simulink model "WR_UDE"  (R2020a)
settings: Solver=ode4  StartTime=0.0  StopTime=tstop  FixedStep=tstep  RelTol=1e-3
values from neighbouring files (symbols this model uses):
  eic = xic - xmic    [data.m]
  K = dlqr(F_n, G_n, Q, R)    [data.m]
  Ts = 0.01    [data.m]
  udic = (-Ts/T)*pinv(G_n)*eic    [data.m]
  xhat_ic = [pi/9; 0]    [data.m]
  xic = [pi/9; 0]    [data.m]
  xmic = [0; 0]    [data.m]
settings Model: Creator=Ram Padmanabhan  LastModifiedBy=Maithili Shetty
settings DataIOCC: SaveOutput=off  SignalLogging=off  DSMLogging=off  SaveTime=off  ReturnWorkspaceOutputs=off

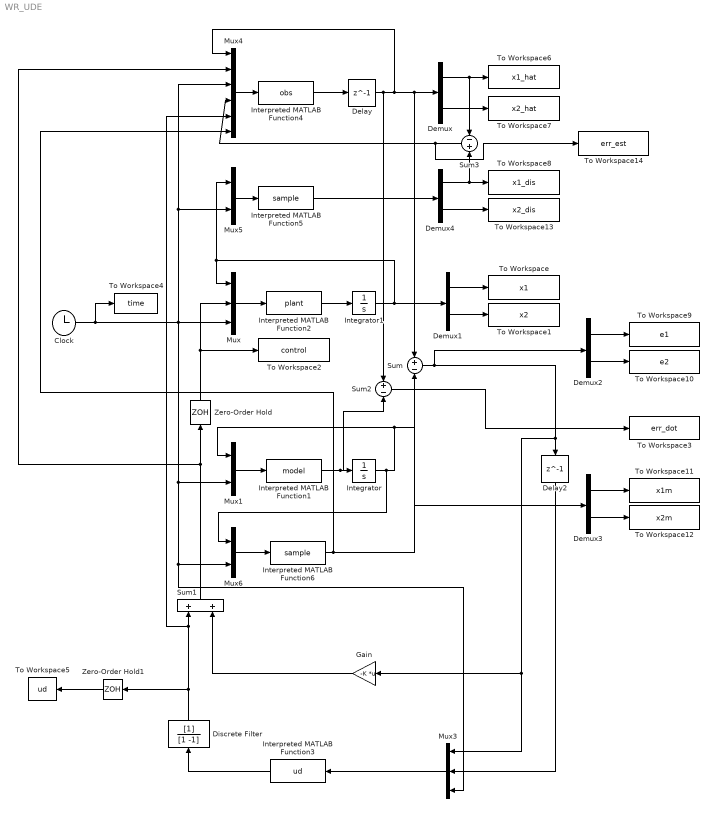
== system WR_UDE ==
  Clock : Clock
  Delay : Delay  DelayLength=1  InitialCondition=xhat_ic  SampleTime=Ts
  Delay2 : Delay  DelayLength=1  InitialCondition=eic  SampleTime=Ts
  Demux{,1..4} (5 alike) : Demux  Outputs=2
  Discrete Filter : DiscreteFilter  Denominator=[1 -1]  InitialStates=udic  SampleTime=Ts
  Gain : Gain  Gain=-K  Multiplication=Matrix(K*u)
  Integrator : Integrator  InitialCondition=xmic
  Integrator1 : Integrator  InitialCondition=xic
  Interpreted MATLAB Function1 : MATLABFcn  MATLABFcn=model  OutputDimensions=2
  Interpreted MATLAB Function2 : MATLABFcn  MATLABFcn=plant  OutputDimensions=2
  Interpreted MATLAB Function3 : MATLABFcn  MATLABFcn=ud  OutputDimensions=1
  Interpreted MATLAB Function4 : MATLABFcn  MATLABFcn=obs  OutputDimensions=2
  Interpreted MATLAB Function5 : MATLABFcn  MATLABFcn=sample  OutputDimensions=2
  Interpreted MATLAB Function6 : MATLABFcn  MATLABFcn=sample  OutputDimensions=2
  Mux : Mux  Inputs=3
  Mux1 : Mux  Inputs=2
  Mux3 : Mux  Inputs=3
  Mux4 : Mux  Inputs=6
  Mux5 : Mux  Inputs=2
  Mux6 : Mux  Inputs=2
  Sum : Sum  Inputs=+-
  Sum1 : Sum
  Sum2 : Sum  Inputs=+-
  Sum3 : Sum  Inputs=-+
  To Workspace : ToWorkspace  VariableName=x1  SampleTime=-1
  To Workspace1 : ToWorkspace  VariableName=x2  SampleTime=-1
  To Workspace10 : ToWorkspace  VariableName=e2  SampleTime=-1
  To Workspace11 : ToWorkspace  VariableName=x1m  SampleTime=-1
  To Workspace12 : ToWorkspace  VariableName=x2m  SampleTime=-1
  To Workspace13 : ToWorkspace  VariableName=x2_dis  SampleTime=-1
  To Workspace14 : ToWorkspace  VariableName=err_est  SampleTime=Ts
  To Workspace2 : ToWorkspace  VariableName=control  SampleTime=-1
  To Workspace3 : ToWorkspace  VariableName=err_dot  SampleTime=-1
  To Workspace4 : ToWorkspace  VariableName=time  SampleTime=-1
  To Workspace5 : ToWorkspace  VariableName=ud  SampleTime=-1
  To Workspace6 : ToWorkspace  VariableName=x1_hat  SampleTime=-1
  To Workspace7 : ToWorkspace  VariableName=x2_hat  SampleTime=-1
  To Workspace8 : ToWorkspace  VariableName=x1_dis  SampleTime=-1
  To Workspace9 : ToWorkspace  VariableName=e1  SampleTime=-1
  Zero-Order Hold : ZeroOrderHold  SampleTime=Ts
  Zero-Order Hold1 : ZeroOrderHold  SampleTime=Ts
  wires:
  Sum/1 -> Delay2/1, Mux3/1, Gain/1, Demux2/1
  Mux5/1 -> Interpreted MATLAB Function5/1
  Interpreted MATLAB Function5/1 -> Demux4/1
  Sum2/1 -> To Workspace3/1
  Gain/1 -> Sum1/2
  Demux/1 -> Sum3/1, To Workspace6/1
  Demux/2 -> To Workspace7/1
  Zero-Order Hold/1 -> To Workspace2/1, Mux/2
  Zero-Order Hold1/1 -> To Workspace5/1
  Demux1/1 -> To Workspace/1
  Demux3/1 -> To Workspace11/1
  Demux2/2 -> To Workspace10/1
  Interpreted MATLAB Function2/1 -> Integrator1/1
  Demux1/2 -> To Workspace1/1
  Mux1/1 -> Interpreted MATLAB Function1/1
  Discrete Filter/1 -> Mux4/5, Sum1/1, Zero-Order Hold1/1
  Clock/1 -> Mux5/2, Mux4/3, Mux6/2, Mux3/3, Mux1/2, Mux/3, To Workspace4/1
  Interpreted MATLAB Function3/1 -> Discrete Filter/1
  Demux3/2 -> To Workspace12/1
  Integrator1/1 -> Demux1/1, Mux5/1, Mux/1
  Interpreted MATLAB Function1/1 -> Sum2/2, Integrator/1
  Mux/1 -> Interpreted MATLAB Function2/1
  Sum1/1 -> Mux4/2, Zero-Order Hold/1
  Sum3/1 -> To Workspace14/1, Mux4/4
  Interpreted MATLAB Function4/1 -> Delay/1
  Mux6/1 -> Interpreted MATLAB Function6/1
  Demux4/2 -> To Workspace13/1
  Integrator/1 -> Mux6/1, Demux3/1, Mux1/1
  Delay2/1 -> Mux3/2
  Delay/1 -> Mux4/1, Sum/1, Demux/1, Sum2/1
  Mux3/1 -> Interpreted MATLAB Function3/1
  Demux4/1 -> Sum3/2, To Workspace8/1
  Mux4/1 -> Interpreted MATLAB Function4/1
  Demux2/1 -> To Workspace9/1
  Interpreted MATLAB Function6/1 -> Mux4/6, Sum/2
